simulink model "XY_2mm_accelcontrol"  (R2023a)
settings: Solver=ode1  StartTime=0.0  StopTime=inf  FixedStep=0.001  RelTol=1e-3  EnableMultiTasking=on
PostLoadFcn:
  | , if any(exist('dsrtsu_mdlpostloadfcn', 'file') ~= 0), dsrtsu_mdlpostloadfcn('Execute', bdroot); end,
InitFcn:
  | , if any(exist('rtifpga_mdlclblib', 'file') ~= 0), rtifpga_mdlclblib('Init', bdroot); end,
  | [b,a] = butter(6,0.6)
  | N_coils = 6
  | % Load mean voltage needed for stationary levitation at "center" for the ML model's given dataset
  | load("D:\Maglev_Project\00_WORKSTATION\MATLAB Training\alldata.mat","Vmean_raw")
  | tic
model workspace (MAT data in the model file):
  Iters = 5
  N_coils = 6
  fatness_default = 1
  running = 0
  z0_default = 0.080001
undefined symbols (not defined in the file or in its folder): a, b, DiscIntNeverNeededParam, Vmean_raw
libraries: neural x15, simulink x8, commfilt2 x7, dspstat3 x4, rti2004lib x3, rtilibm x1
(part 2 of 3)

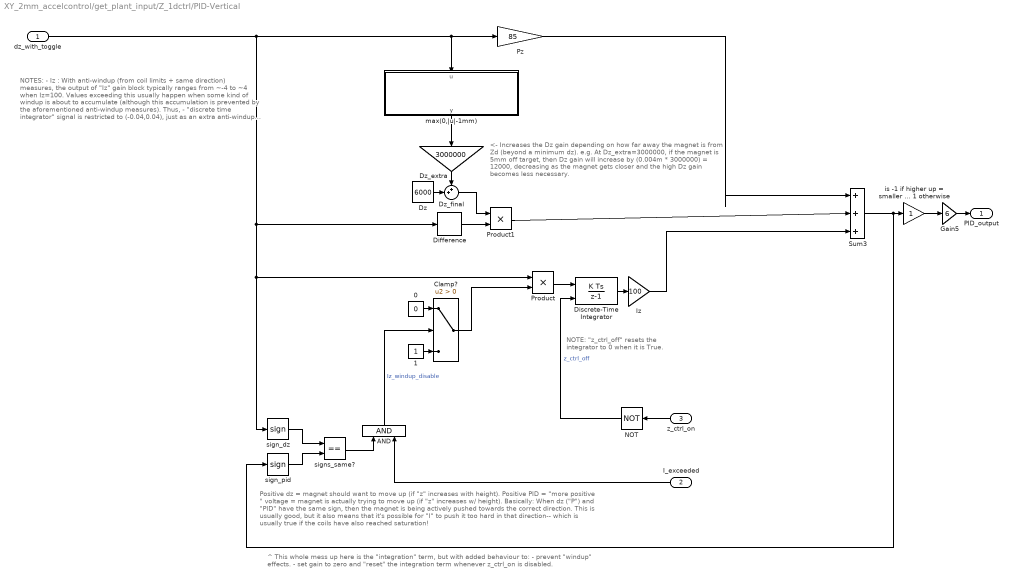
== system XY_2mm_accelcontrol/get_plant_input/Z_1dctrl/PID-Vertical ==
  note: <- Increases the Dz gain depending on how far away the magnet is from Zd (beyond a minimum dz).
      | e.g. At Dz_extra=3000000, if the magnet is 5mm off target, then Dz gain will increase by (0.004m * 3000000) = 12000, decreasing as the magnet gets closer and the high Dz gain becomes less necessary.
  note: NOTE: "z_ctrl_off" resets the integrator to 0 when it is True.
  note: NOTES:
      | - Iz : With anti-windup (from coil limits + same direction) measures, the output of "Iz" gain block typically ranges from ~-4 to ~4 when Iz=100. Values exceeding this usually happen when some kind of windup is about to accumulate (although this accumulation is prevented by the aforementioned anti-windup measures).
      | Thus,
      | - "discrete time integrator" signal is restricted to (-0.04,0.04), just as an extra anti-windup measure.
      | - Also, the integral resets while z-control is disabled.
  note: ^ This whole mess up here is the "integration" term, but with added behaviour to:
      | - prevent "windup" effects.
      | - set gain to zero and "reset" the integration term whenever z_ctrl_on is disabled.
  note: Positive dz = magnet should want to move up (if "z" increases with height).
      | Positive PID = "more positive " voltage = magnet is actually trying to move up (if "z" increases w/ height).
      |
      | Basically: When dz ("P") and "PID" have the same sign, then the magnet is being actively pushed towards the correct direction. This is usually good, but it also means that it's possible for "I" to push it too hard in that direction-- which is usually true if the coils have also reached saturation!
  dz_with_toggle : Inport
  I_exceeded : Inport  Port=2
  z_ctrl_on : Inport  Port=3
  0 : Constant  Value=0
  1 : Constant
  AND : Logic  AllPortsSameDT=off  OutDataTypeStr=boolean
  Clamp? : Switch  Criteria=u2 > Threshold  SaturateOnIntegerOverflow=off  InputSameDT=off
  Difference : simulink/Discrete/Difference  ICPrevInput=0.0  OutMin=[]  OutMax=[]  OutDataType=fixdt(1, 16)  OutScaling=2^-10  DoSatur=off
  Discrete-Time Integrator : DiscreteIntegrator  ExternalReset=sampled level  SampleTime=-1  LimitOutput=on  UpperSaturationLimit=0.04  LowerSaturationLimit=-0.04  ICPrevOutput=DiscIntNeverNeededParam  ICPrevScaledInput=DiscIntNeverNeededParam
  Dz : Constant  Value=6000
  Dz_extra : Gain  Gain=3000000
  Dz_final : Sum  Inputs=++|
  Gain5 : Gain  Gain=6
  Iz : Gain  Gain=100
  NOT : Logic  Operator=NOT  AllPortsSameDT=off  OutDataTypeStr=boolean
  Product : Product
  Product1 : Product
  Pz : Gain  Gain=85
  Sum3 : Sum  Inputs=|+++
  "is -1 if higher up = smaller z, 1 otherwise" : Gain
  max(0,|u|-1mm) : MATLAB Function  TreatAsAtomicUnit=on
  sign_dz : Signum
  sign_pid : Signum
  signs_same? : RelationalOperator  Operator===  OutDataTypeStr=boolean  RndMeth=Simplest  InputSameDT=off
  PID_output : Outport
  wires:
  Pz/1 -> Sum3/1
  Difference/1 -> Product1/2
  Product1/1 -> Sum3/2
  Sum3/1 -> sign_pid/1, "is -1 if higher up = smaller z, 1 otherwise"/1
  "is -1 if higher up = smaller z, 1 otherwise"/1 -> Gain5/1
  Gain5/1 -> PID_output/1
  0/1 -> Clamp?/1
  Discrete-Time Integrator/1 -> Iz/1
  Clamp?/1 -> Product/2
  Product/1 -> Discrete-Time Integrator/1
  1/1 -> Clamp?/3
  sign_dz/1 -> signs_same?/1
  sign_pid/1 -> signs_same?/2
  signs_same?/1 -> AND/1
  I_exceeded/1 -> AND/2
  AND/1 -> Clamp?/2  "Iz_windup_disable"
  z_ctrl_on/1 -> NOT/1
  NOT/1 -> Discrete-Time Integrator/2  "z_ctrl_off"
  Iz/1 -> Sum3/3
  dz_with_toggle/1 -> Difference/1, sign_dz/1, Product/1, max(0,|u|-1mm)/1(u), Pz/1
  Dz/1 -> Dz_final/2
  max(0,|u|-1mm)/1(y) -> Dz_extra/1
  Dz_extra/1 -> Dz_final/1
  Dz_final/1 -> Product1/1

== system XY_2mm_accelcontrol/get_plant_input/acceleration_to_I_ratio/Actually apply voltages ==
  note: Behaviour summary:
      | (HOLD, START):
      | 	(ON, ON)	- Voltage ratio is updated, but then stays constant
      | 	(ON, OFF)	- Voltage ratio cannot change
      |
      | 	(OFF, ON)	- Voltage ratio is continually updated to maintain input acceleration
      | 	(OFF, OFF)	- Voltage ratio cannot change
  note: User inputs:
      | “Hold ratio”
      | ON: Voltage ratio is held, so magnet will (ideally) accelerate as specified VERY BRIEFLY before settling at a Bmax point
      | OFF: Voltage ratio is dynamically adjusted to maintain the input acceleration (i.e. magnet will speed up endlessly)
      |
      | "Start acceleration" (HOLD)
      | ON: Voltage ratio is allowed to change while pressed
      | OFF: Voltage ratio is NOT allowed to change
  Voltages : Inport
  Hold ratio : Constant
  Start Acceleration : Constant  Value=0
  allow_voltage_update : Subsystem
  voltages_updated : Subsystem  TreatAsAtomicUnit=on
  Out1 : Outport
  wires:
  voltages_updated/1(voltages_updated) -> Out1/1
  Hold ratio/1 -> allow_voltage_update/1(Hold)
  Voltages/1 -> voltages_updated/1(voltages)
  Start Acceleration/1 -> allow_voltage_update/2(Start)
  allow_voltage_update/1(allow_voltage_update) -> voltages_updated/Enable

== system XY_2mm_accelcontrol/get_plant_input/acceleration_to_I_ratio/Make ratios add up to 1 ==
  note: Modified coil ratio distribution is ""normalized"" (NOT vector normalization) such that its sum equals 1.
  Voltages : Inport
  Divide : Product  Inputs=*/
  Sum of Elements : Sum  Inputs=+
  Voltage_ratio : Outport
  wires:
  Voltages/1 -> Sum of Elements/1, Divide/1
  Sum of Elements/1 -> Divide/2
  Divide/1 -> Voltage_ratio/1

== system XY_2mm_accelcontrol/get_plant_input/acceleration_to_I_ratio/Voltages from ML ==
  note: Current ML model (" DEFAULT_goodunits_filtervolts_TEMP ") inputs XY position (in mm) and a desired XY acceleration (in mm/s/s), and outputs final input voltages (i.e. voltages fed into amplifier) in V.
  xy_acc_mmss : Inport
  xy_mm : Inport  Port=2
  Function Fitting Neural Network : Subsystem
      mask help: Function Fitting Neural Network
      mask Display: e = 0.06;c1 = [120 150 230]/255;c2 = ([120 150 230]+0)/383;c3 = ([120 150 230]+128)/383;patch([0 1 1 0],[0 0 1 1],c1);patch([0 1 1 1-e 1-e 0+e],[0 0 1 1-e 0+e 0+e],c2);patch([0 0 1 1-e 0+e 0+e],[0 1 1 1-e 1-e 0+e],c3);plot([0 1 1 0 0],[0 0 1 1 0]);fprintf('NNET');port_label('input',1,' Input');port_label('output',1,'Output ');
  Mux : Mux  Inputs=2
  Sum : Sum  Inputs=|++
  Vmean : Constant  Value=Vmean_raw
  Voltages : Outport
  wires:
  xy_acc_mmss/1 -> Mux/2
  Vmean/1 -> Sum/2
  Function Fitting Neural Network/1(Output) -> Sum/1
  Sum/1 -> Voltages/1
  xy_mm/1 -> Mux/1
  Mux/1 -> Function Fitting Neural Network/1(Input)

== system XY_2mm_accelcontrol/get_plant_input/choose_Z_d_temp/istrue_for_X_time ==
  note: When is nonzero or true , the integrator accumulates by 1 per cycle. The counter stops and resets to 0 whenever input==0. Once the integrator crosses a certain threshold , the subsystem outputs 1 (0 otherwise). (In other words, it's just a timer for how long " logical(input) == 1 " has been maintained.)
      |
      | Basically, this subsystem outputs 1 if the input signal has been nonzero for X amount of time. Otherwise, it outputs 0.
  input : Inport
  Data Type Conversion : DataTypeConversion  OutDataTypeStr=boolean  SaturateOnIntegerOverflow=off  RndMeth=Floor
  Discrete-Time Accumulator (ms) : DiscreteIntegrator  IntegratorMethod=Accumulation: Forward Euler  ExternalReset=sampled level  SampleTime=-1  OutDataTypeStr=double  ICPrevOutput=DiscIntNeverNeededParam  ICPrevScaledInput=DiscIntNeverNeededParam
  GreaterThan : RelationalOperator  Operator=>  OutDataTypeStr=boolean  RndMeth=Simplest  InputSameDT=off
  NOT : Logic  Operator=NOT  AllPortsSameDT=off  OutDataTypeStr=boolean
  threshold_ms : Constant  Value=500
  input_held : Outport
  wires:
  input/1 -> Data Type Conversion/1
  Discrete-Time Accumulator (ms)/1 -> GreaterThan/1
  threshold_ms/1 -> GreaterThan/2
  NOT/1 -> Discrete-Time Accumulator (ms)/2
  GreaterThan/1 -> input_held/1
  Data Type Conversion/1 -> NOT/1, Discrete-Time Accumulator (ms)/1

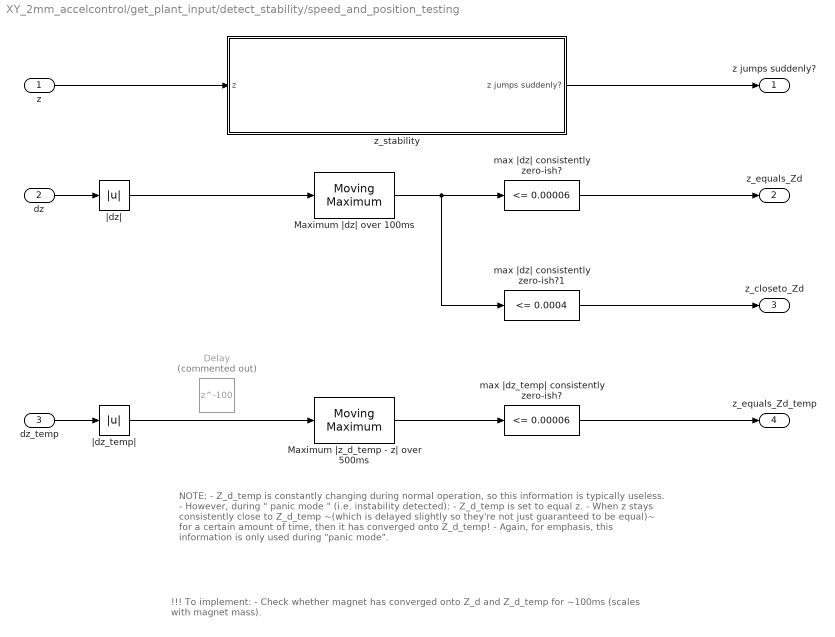
== system XY_2mm_accelcontrol/get_plant_input/detect_stability/speed_and_position_testing ==
  note: !!! To implement:
      | - Check whether magnet has converged onto Z_d and Z_d_temp for ~100ms (scales with magnet mass).
  note: NOTE:
      | - Z_d_temp is constantly changing during normal operation, so this information is typically useless.
      | - However, during " panic mode " (i.e. instability detected):
      | - Z_d_temp is set to equal z.
      | - When z stays consistently close to Z_d_temp ~(which is delayed slightly so they're not just
      | guaranteed to be equal)~ for a certain amount of time, then it has converged onto Z_d_temp!
      | - Again, for emphasis, this information is only used during "panic mode".
  z : Inport
  dz : Inport  Port=2
  dz_temp : Inport  Port=3
  Delay : Delay  Commented=on  DelayLength=100
  Maximum |dz| over 100ms : dspstat3/Moving Maximum  SpecifyWindowLength=on  WindowLength=100  SimulateUsing=Code generation
  Maximum |z_d_temp - z| over 500ms : dspstat3/Moving Maximum  SpecifyWindowLength=on  WindowLength=500  SimulateUsing=Code generation
  max |dz_temp| consistently zero-ish? : simulink/Logic and Bit Operations/Compare To Constant  relop=<=  const=0.00006  OutDataTypeStr=boolean
  max |dz| consistently zero-ish? : simulink/Logic and Bit Operations/Compare To Constant  relop=<=  const=0.00006  OutDataTypeStr=boolean
  max |dz| consistently zero-ish?1 : simulink/Logic and Bit Operations/Compare To Constant  relop=<=  const=0.0004  OutDataTypeStr=boolean
  z_stability : Subsystem
  |dz_temp| : Abs  SaturateOnIntegerOverflow=off
  |dz| : Abs  SaturateOnIntegerOverflow=off
  z jumps suddenly? : Outport
  z_equals_Zd : Outport  Port=2
  z_closeto_Zd : Outport  Port=3
  z_equals_Zd_temp : Outport  Port=4
  wires:
  |dz|/1 -> Maximum |dz| over 100ms/1
  max |dz| consistently zero-ish?/1 -> z_equals_Zd/1
  dz/1 -> |dz|/1
  Maximum |z_d_temp - z| over 500ms/1 -> max |dz_temp| consistently zero-ish?/1
  max |dz_temp| consistently zero-ish?/1 -> z_equals_Zd_temp/1
  dz_temp/1 -> |dz_temp|/1
  |dz_temp|/1 -> Maximum |z_d_temp - z| over 500ms/1
  z/1 -> z_stability/1(z)
  max |dz| consistently zero-ish?1/1 -> z_closeto_Zd/1
  Maximum |dz| over 100ms/1 -> max |dz| consistently zero-ish?1/1, max |dz| consistently zero-ish?/1
  z_stability/1(z jumps suddenly?) -> z jumps suddenly?/1

== system XY_2mm_accelcontrol/plant/Position Determination1/10ms mean x ==
  note: NOTE: Sensor readings fluctuate over a peak-to-peak amplitude of about 4.5e-5 m, over a period of almost exactly 10ms.
      |
      | 08/14/23: See how it improves if I only consider the mean signal over 10ms!
  In1 : Inport
  ave signal : Product  Inputs=*/
  integration window (samples) : Constant  Value=10
  sum of signal over short time : commfilt2/Windowed Integrator  integperiod=10  InputProcessing=Columns as channels (frame based)  roundingMode=Floor  overflowMode=off  coeffDataTypeStr=Inherit: Same word length as input  coeffMin=[]  coeffMax=[]  coeffLastDataTypeStr=Inherit: Same word length as input  accumDataTypeStr=Inherit: Same as product output  accumLastDataTypeStr=Inherit: Same as product output  outputDataTypeStr=Inherit: Same as accumulator  outputMin=[]  outputMax=[]  outputLastDataTypeStr=Inherit: Same as accumulator
  X(m) : Outport
  wires:
  sum of signal over short time/1 -> ave signal/1
  In1/1 -> sum of signal over short time/1
  integration window (samples)/1 -> ave signal/2
  ave signal/1 -> X(m)/1

== system XY_2mm_accelcontrol/plant/Position Determination1/10ms mean y ==
  note: NOTE: Sensor readings fluctuate over a peak-to-peak amplitude of about 4.5e-5 m, over a period of almost exactly 10ms.
      |
      | 08/14/23: See how it improves if I only consider the mean signal over 10ms!
  In1 : Inport
  ave signal : Product  Inputs=*/
  integration window (samples) : Constant  Value=10
  sum of signal over short time : commfilt2/Windowed Integrator  integperiod=10  InputProcessing=Columns as channels (frame based)  roundingMode=Floor  overflowMode=off  coeffDataTypeStr=Inherit: Same word length as input  coeffMin=[]  coeffMax=[]  coeffLastDataTypeStr=Inherit: Same word length as input  accumDataTypeStr=Inherit: Same as product output  accumLastDataTypeStr=Inherit: Same as product output  outputDataTypeStr=Inherit: Same as accumulator  outputMin=[]  outputMax=[]  outputLastDataTypeStr=Inherit: Same as accumulator
  Y(m) : Outport
  wires:
  sum of signal over short time/1 -> ave signal/1
  In1/1 -> sum of signal over short time/1
  integration window (samples)/1 -> ave signal/2
  ave signal/1 -> Y(m)/1

== system XY_2mm_accelcontrol/plant/Position Determination1/10ms mean z ==
  note: NOTE: Sensor readings fluctuate over a peak-to-peak amplitude of about 4.5e-5 m, over a period of almost exactly 10ms.
      |
      | 08/14/23: See how it improves if I only consider the mean signal over 10ms!
  In1 : Inport
  ave signal : Product  Inputs=*/
  integration window (samples) : Constant  Value=10
  sum of signal over short time : commfilt2/Windowed Integrator  integperiod=10  InputProcessing=Columns as channels (frame based)  roundingMode=Floor  overflowMode=off  coeffDataTypeStr=Inherit: Same word length as input  coeffMin=[]  coeffMax=[]  coeffLastDataTypeStr=Inherit: Same word length as input  accumDataTypeStr=Inherit: Same as product output  accumLastDataTypeStr=Inherit: Same as product output  outputDataTypeStr=Inherit: Same as accumulator  outputMin=[]  outputMax=[]  outputLastDataTypeStr=Inherit: Same as accumulator
  Z(m) : Outport
  wires:
  sum of signal over short time/1 -> ave signal/1
  In1/1 -> sum of signal over short time/1
  integration window (samples)/1 -> ave signal/2
  ave signal/1 -> Z(m)/1

== system XY_2mm_accelcontrol/plant/Position Determination1/XY position Calculation ==
  note: !!MODIFIED!!
      | Before: "X_p, Y_p = Head2_read, Head3_read - radius_m".
      | After: "Head2_p, Head3_p = Head2_read, Head3_read + radius_m".
  note: Laser sensors output a voltage in [-10,10]V, proportional to the detected object's position-- which ranges from 0mm (up, given by 10V) to 40mm (down, given by -10V). Size of the object is not taken into account.
  Head II (Voltage) : Inport
  Head III (Voltage) : Inport  Port=2
  diameter_m : Inport  Port=3
  Gain : Gain  Gain=1/2
  Gain2 : Gain  Gain=2/1000
  Gain4 : Gain  Gain=2/1000
  Mux : Mux  Inputs=2
  Sum : Sum  Inputs=|++
  Sum1 : Sum  Inputs=++|
  X_m : Fcn  Expr=(u(1)+u(2))*sin(pi/4)
  Y_m : Fcn  Expr=(u(1)-u(2))*sin(pi/4)
  X_Position(m) : Outport
  Y_Position(m) : Outport  Port=2
  wires:
  Head III (Voltage)/1 -> Gain4/1
  Y_m/1 -> Y_Position(m)/1
  X_m/1 -> X_Position(m)/1
  Head II (Voltage)/1 -> Gain2/1
  Mux/1 -> Y_m/1, X_m/1
  Sum1/1 -> Mux/2  "Head3_p"
  Gain4/1 -> Sum1/2
  Sum/1 -> Mux/1  "Head2_p"
  Gain/1 -> Sum1/1, Sum/2  "radius_m"
  Gain2/1 -> Sum/1
  diameter_m/1 -> Gain/1

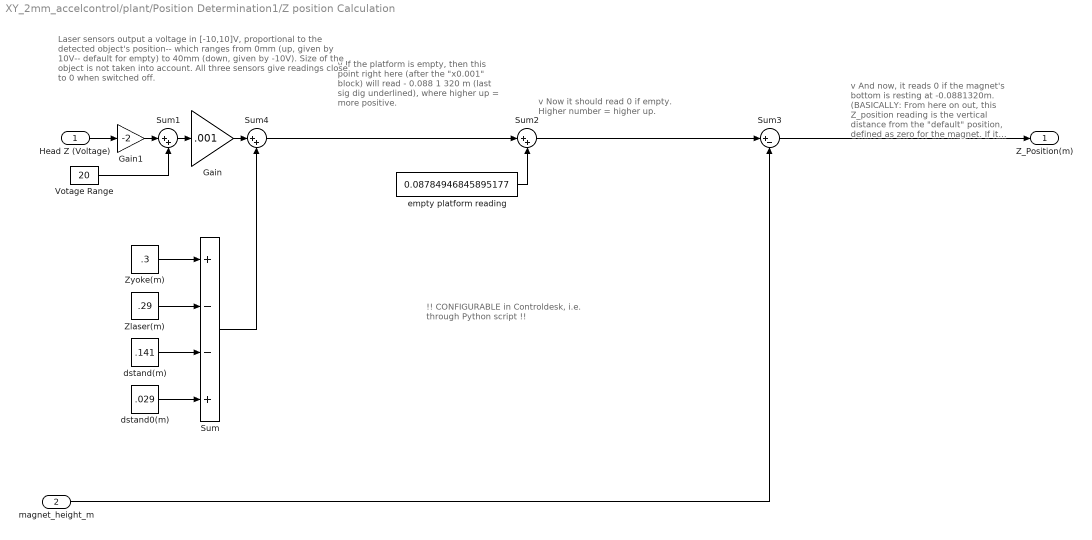
== system XY_2mm_accelcontrol/plant/Position Determination1/Z position Calculation ==
  note: v If the platform is empty, then this point right here (after the "x0.001" block) will read - 0.088 1 320 m (last sig dig underlined), where higher up = more positive.
  note: Laser sensors output a voltage in [-10,10]V, proportional to the detected object's position-- which ranges from 0mm (up, given by 10V-- default for empty) to 40mm (down, given by -10V). Size of the object is not taken into account.
      | All three sensors give readings close to 0 when switched off.
  note: v Now it should read 0 if empty.
      | Higher number = higher up.
  note: v And now, it reads 0 if the magnet's bottom is resting at -0.0881320m.
      |
      | (BASICALLY: From here on out, this Z_position reading is the vertical distance from the "default" position, defined as zero for the magnet. If it reads something significantly different from 0, then double check the magnet height.)
  note: !! CONFIGURABLE in Controldesk, i.e. through Python script !!
  Head Z (Voltage) : Inport
  magnet_height_m : Inport  Port=2
  Gain : Gain  Gain=.001
  Gain1 : Gain  Gain=-2
  Sum : Sum  Inputs=+--+
  Sum1 : Sum  Inputs=|++
  Sum2 : Sum  Inputs=|++
  Sum3 : Sum  Inputs=|+-
  Sum4 : Sum  Inputs=|++
  Votage Range : Constant  Value=20
  Zlaser(m) : Constant  Value=.29
  Zyoke(m) : Constant  Value=.3
  dstand(m) : Constant  Value=.141
  dstand0(m) : Constant  Value=.029
  empty platform reading : Constant  Value=0.08784946845895177
  Z_Position(m) : Outport
  wires:
  Sum2/1 -> Sum3/1
  Head Z (Voltage)/1 -> Gain1/1
  Sum/1 -> Sum4/2
  Sum1/1 -> Gain/1
  Votage Range/1 -> Sum1/2
  Gain1/1 -> Sum1/1
  Zlaser(m)/1 -> Sum/2
  Zyoke(m)/1 -> Sum/1
  dstand(m)/1 -> Sum/3
  dstand0(m)/1 -> Sum/4
  magnet_height_m/1 -> Sum3/2
  Sum4/1 -> Sum2/1
  Gain/1 -> Sum4/1
  empty platform reading/1 -> Sum2/2
  Sum3/1 -> Z_Position(m)/1

== system XY_2mm_accelcontrol/RTI Data/RTI Data Store/RTI Data Store/RTI Data Store ==
  RTI Data Store : Subsystem  mask(RTI_DATA_STORE){}
      mask help:
      | RTI Data Store Block. This block is used by RTI to store internal model dependent data. Deleting this block will result in data loss.
      |
      | NEVER DELETE, COPY, OR MODIFY THIS BLOCK!
      mask Help:
      | RTI Data Store Block. This block is used by RTI to store internal model dependent data. Deleting this block will result in data loss.
      | 
      | NEVER DELETE, COPY, OR MODIFY THIS BLOCK!
      mask Display: text(0.5, 0.5, ' ', 'HorizontalAlignment', 'center');

== system XY_2mm_accelcontrol/get_plant_input/acceleration_to_I_ratio/Actually apply voltages/allow_voltage_update ==
  Hold : Inport
  Start : Inport  Port=2
  AND : Logic  AllPortsSameDT=off  OutDataTypeStr=boolean
  NOT : Logic  Operator=NOT  IconShape=distinctive  AllPortsSameDT=off  OutDataTypeStr=boolean
  OR : Logic  Operator=OR  AllPortsSameDT=off  OutDataTypeStr=boolean
  was Start just enabled : Subsystem
  allow_voltage_update : Outport
  wires:
  Start/1 -> was Start just enabled/1(Start), AND/2
  Hold/1 -> NOT/1
  AND/1 -> allow_voltage_update/1
  was Start just enabled/1(just_activated) -> OR/2
  OR/1 -> AND/1
  NOT/1 -> OR/1

== system XY_2mm_accelcontrol/get_plant_input/acceleration_to_I_ratio/Actually apply voltages/voltages_updated ==
  voltages : Inport
  Enable : EnablePort
  voltages_updated : Outport
  wires:
  voltages/1 -> voltages_updated/1

== system XY_2mm_accelcontrol/get_plant_input/acceleration_to_I_ratio/Voltages from ML/Function Fitting Neural Network ==
  Input : Inport  PortDimensions=4
      mask Display: e = 0.06;c1 = [120 230 180]/255;c2 = ([120 230 180]+0)/(256+128);c3 = ([120 230 180]+128)/(256+128);patch([0 1 1 0],[0 0 1 1],c1);patch([0 1 1 1-e 1-e 0+e],[0 0 1 1-e 0+e 0+e],c2);patch([0 0 1 1-e 0+e 0+e],[0 1 1 1-e 1-e 0+e],c3);plot([0 1 1 0 0],[0 0 1 1 0]);
  Layer 1 : Subsystem
      mask Display: e = 0.06;c1 = [120 150 230]/255;c2 = ([120 150 230]+0)/383;c3 = ([120 150 230]+128)/383;patch([0 1 1 0],[0 0 1 1],c1);patch([0 1 1 1-e 1-e 0+e],[0 0 1 1-e 0+e 0+e],c2);patch([0 0 1 1-e 0+e 0+e],[0 1 1 1-e 1-e 0+e],c3);plot([0 1 1 0 0],[0 0 1 1 0]);
  Layer 2 : Subsystem
      mask Display: e = 0.06;c1 = [120 150 230]/255;c2 = ([120 150 230]+0)/383;c3 = ([120 150 230]+128)/383;patch([0 1 1 0],[0 0 1 1],c1);patch([0 1 1 1-e 1-e 0+e],[0 0 1 1-e 0+e 0+e],c2);patch([0 0 1 1-e 0+e 0+e],[0 1 1 1-e 1-e 0+e],c3);plot([0 1 1 0 0],[0 0 1 1 0]);
  Process Input 1 : Subsystem
      mask Display: e = 0.06;c1 = [120 150 230]/255;c2 = ([120 150 230]+0)/383;c3 = ([120 150 230]+128)/383;patch([0 1 1 0],[0 0 1 1],c1);patch([0 1 1 1-e 1-e 0+e],[0 0 1 1-e 0+e 0+e],c2);patch([0 0 1 1-e 0+e 0+e],[0 1 1 1-e 1-e 0+e],c3);plot([0 1 1 0 0],[0 0 1 1 0]);
  Process Output 1 : Subsystem
      mask Display: e = 0.06;c1 = [120 150 230]/255;c2 = ([120 150 230]+0)/383;c3 = ([120 150 230]+128)/383;patch([0 1 1 0],[0 0 1 1],c1);patch([0 1 1 1-e 1-e 0+e],[0 0 1 1-e 0+e 0+e],c2);patch([0 0 1 1-e 0+e 0+e],[0 1 1 1-e 1-e 0+e],c3);plot([0 1 1 0 0],[0 0 1 1 0]);
  Output : Outport  InitialOutput=[0;0;0;0;0;0]
      mask Display: e = 0.06;c1 = [120 230 180]/255;c2 = ([120 230 180]+0)/(256+128);c3 = ([120 230 180]+128)/(256+128);patch([0 1 1 0],[0 0 1 1],c1);patch([0 1 1 1-e 1-e 0+e],[0 0 1 1-e 0+e 0+e],c2);patch([0 0 1 1-e 0+e 0+e],[0 1 1 1-e 1-e 0+e],c3);plot([0 1 1 0 0],[0 0 1 1 0]);
  wires:
  Input/1 -> Process Input 1/1(x)
  Process Output 1/1(y) -> Output/1
  Process Input 1/1(p) -> Layer 1/1("p{1}")
  Layer 1/1("a{1}") -> [feedback1]
  [feedback1] -> Layer 2/1("a{1} ")
  Layer 2/1("a{2}") -> Process Output 1/1(a)

== system XY_2mm_accelcontrol/get_plant_input/detect_stability/speed_and_position_testing/z_stability ==
  note: NOTE:
      | When Zd changes, the speed peaks spike up from ~5e-7m/s to around ~2e-5 m/s.
      |
      | When the magnet struggles to converge, the speed peaks spike up to ~1e-5 or more.
      |
      | Thus: 0.5e-5 m/s seems to be a good line beyond which speed peaks indicate either intentional vertical movement OR struggle/failure to converge onto Zd. When this occurs will be tracked using a moving maximum over some short timeframe (~100ms?).
      |
      | ** The above is WITH "z" being the 10ms average of the raw signal. Changing this may require recalibration of this speed threshold. **
  z : Inport
  Abs : Abs  Commented=on  SaturateOnIntegerOverflow=off
  Highest z in past 25ms : dspstat3/Moving Maximum  Commented=on  SpecifyWindowLength=on  WindowLength=25  SimulateUsing=Code generation
  Lowest z in past 25ms : dspstat3/Moving Minimum  Commented=on  SpecifyWindowLength=on  WindowLength=25  SimulateUsing=Code generation
  Sum : Sum  Commented=on  Inputs=|+-|
  ave z : Product  Inputs=*/
  average |z - z_prev|/dt (m/ms) too high? : simulink/Logic and Bit Operations/Compare To Constant  relop=>=  const=0.5e-5  OutDataTypeStr=boolean
  integration window (samples)2 : Constant  Value=10
  sum of z over 10ms1 : commfilt2/Windowed Integrator  integperiod=10  InputProcessing=Columns as channels (frame based)  roundingMode=Floor  overflowMode=off  coeffDataTypeStr=Inherit: Same word length as input  coeffMin=[]  coeffMax=[]  coeffLastDataTypeStr=Inherit: Same word length as input  accumDataTypeStr=Inherit: Same as product output  accumLastDataTypeStr=Inherit: Same as product output  outputDataTypeStr=Inherit: Same as accumulator  outputMin=[]  outputMax=[]  outputLastDataTypeStr=Inherit: Same as accumulator
  z - z_previous : simulink/Discrete/Difference  ICPrevInput=0.0  OutMin=[]  OutMax=[]  OutDataType=fixdt(1, 16)  OutScaling=2^-10  DoSatur=off
  z jumps by more than 0.15mm in 25ms? : simulink/Logic and Bit Operations/Compare To Constant  Commented=on  relop=>=  const=0.00015  OutDataTypeStr=boolean
  |z - z_previous| : Abs  SaturateOnIntegerOverflow=off
  z jumps suddenly? : Outport
  wires:
  Abs/1 -> z jumps by more than 0.15mm in 25ms?/1
  z/1 -> sum of z over 10ms1/1
  Highest z in past 25ms/1 -> Sum/2
  Sum/1 -> Abs/1
  Lowest z in past 25ms/1 -> Sum/1
  z jumps by more than 0.15mm in 25ms?/1 -> ?
  integration window (samples)2/1 -> ave z/2
  sum of z over 10ms1/1 -> ave z/1
  z - z_previous/1 -> |z - z_previous|/1
  ave z/1 -> z - z_previous/1
  |z - z_previous|/1 -> average |z - z_prev|/dt (m/ms) too high?/1
  average |z - z_prev|/dt (m/ms) too high?/1 -> z jumps suddenly?/1

== system XY_2mm_accelcontrol/RTI Data/RTI Data Store/RTI Data Store/RTI Data Store/RTI Data Store ==

== system XY_2mm_accelcontrol/get_plant_input/acceleration_to_I_ratio/Actually apply voltages/allow_voltage_update/was Start just enabled ==
  Start : Inport
  Delay One Step : Delay  DelayLength=1
  Greaterthan : RelationalOperator  Operator=>  OutDataTypeStr=boolean  RndMeth=Simplest  InputSameDT=off
  just_activated : Outport
  wires:
  Start/1 -> Greaterthan/1, Delay One Step/1
  Delay One Step/1 -> Greaterthan/2
  Greaterthan/1 -> just_activated/1

== system XY_2mm_accelcontrol/get_plant_input/acceleration_to_I_ratio/Voltages from ML/Function Fitting Neural Network/Layer 1 ==
  "p{1}" : Inport  PortDimensions=4
      mask Display: e = 0.06;c1 = [120 230 180]/255;c2 = ([120 230 180]+0)/(256+128);c3 = ([120 230 180]+128)/(256+128);patch([0 1 1 0],[0 0 1 1],c1);patch([0 1 1 1-e 1-e 0+e],[0 0 1 1-e 0+e 0+e],c2);patch([0 0 1 1-e 0+e 0+e],[0 1 1 1-e 1-e 0+e],c3);plot([0 1 1 0 0],[0 0 1 1 0]);
  Delays 1 : Subsystem
      mask Display: e = 0.06;c1 = [120 150 230]/255;c2 = ([120 150 230]+0)/383;c3 = ([120 150 230]+128)/383;patch([0 1 1 0],[0 0 1 1],c1);patch([0 1 1 1-e 1-e 0+e],[0 0 1 1-e 0+e 0+e],c2);patch([0 0 1 1-e 0+e 0+e],[0 1 1 1-e 1-e 0+e],c3);plot([0 1 1 0 0],[0 0 1 1 0]);disp('0');
  "IW{1,1}" : Subsystem
      mask Display: e = 0.06;c1 = [120 150 230]/255;c2 = ([120 150 230]+0)/383;c3 = ([120 150 230]+128)/383;patch([0 1 1 0],[0 0 1 1],c1);patch([0 1 1 1-e 1-e 0+e],[0 0 1 1-e 0+e 0+e],c2);patch([0 0 1 1-e 0+e 0+e],[0 1 1 1-e 1-e 0+e],c3);plot([0 1 1 0 0],[0 0 1 1 0]);disp('W');
  "b{1}" : Constant  Value=[0.2425447899040890920030477673208224587142467498779296875;0.99314547038972278425461581718991510570049285888671875;-0.328895397762378915995640227265539579093456268310546875;-1.38849780916554177423449800699017941951751708984375;-0.26530583823266418175279568458790890872478485107421875]
      mask Display: e = 0.06;c1 = [120 150 230]/255;c2 = ([120 150 230]+0)/383;c3 = ([120 150 230]+128)/383;patch([0 1 1 0],[0 0 1 1],c1);patch([0 1 1 1-e 1-e 0+e],[0 0 1 1-e 0+e 0+e],c2);patch([0 0 1 1-e 0+e 0+e],[0 1 1 1-e 1-e 0+e],c3);plot([0 1 1 0 0],[0 0 1 1 0]);disp('b');
  netsum : Sum  Inputs=2  InputSameDT=on  SaturateOnIntegerOverflow=on  OutDataTypeStr=Inherit: Same as first input
      mask Display: e = 0.06;c1 = [120 150 230]/255;c2 = ([120 150 230]+0)/383;c3 = ([120 150 230]+128)/383;patch([0 1 1 0],[0 0 1 1],c1);patch([0 1 1 1-e 1-e 0+e],[0 0 1 1-e 0+e 0+e],c2);patch([0 0 1 1-e 0+e 0+e],[0 1 1 1-e 1-e 0+e],c3);plot([0 1 1 0 0],[0 0 1 1 0]);disp('+');
  tansig : neural/Transfer Functions/tansig
  "a{1}" : Outport  InitialOutput=[0;0;0;0;0]
      mask Display: e = 0.06;c1 = [120 230 180]/255;c2 = ([120 230 180]+0)/(256+128);c3 = ([120 230 180]+128)/(256+128);patch([0 1 1 0],[0 0 1 1],c1);patch([0 1 1 1-e 1-e 0+e],[0 0 1 1-e 0+e 0+e],c2);patch([0 0 1 1-e 0+e 0+e],[0 1 1 1-e 1-e 0+e],c3);plot([0 1 1 0 0],[0 0 1 1 0]);
  wires:
  "p{1}"/1 -> Delays 1/1("p{1}")
  Delays 1/1("pd{1,1}") -> "IW{1,1}"/1("pd{1,1}")
  "IW{1,1}"/1("iz{1,1}") -> netsum/1
  "b{1}"/1 -> netsum/2
  netsum/1 -> tansig/1
  tansig/1 -> "a{1}"/1

== system XY_2mm_accelcontrol/get_plant_input/acceleration_to_I_ratio/Voltages from ML/Function Fitting Neural Network/Layer 2 ==
  "a{1} " : Inport  PortDimensions=5
      mask Display: e = 0.06;c1 = [120 230 180]/255;c2 = ([120 230 180]+0)/(256+128);c3 = ([120 230 180]+128)/(256+128);patch([0 1 1 0],[0 0 1 1],c1);patch([0 1 1 1-e 1-e 0+e],[0 0 1 1-e 0+e 0+e],c2);patch([0 0 1 1-e 0+e 0+e],[0 1 1 1-e 1-e 0+e],c3);plot([0 1 1 0 0],[0 0 1 1 0]);
  Delays 1 : Subsystem
      mask Display: e = 0.06;c1 = [120 150 230]/255;c2 = ([120 150 230]+0)/383;c3 = ([120 150 230]+128)/383;patch([0 1 1 0],[0 0 1 1],c1);patch([0 1 1 1-e 1-e 0+e],[0 0 1 1-e 0+e 0+e],c2);patch([0 0 1 1-e 0+e 0+e],[0 1 1 1-e 1-e 0+e],c3);plot([0 1 1 0 0],[0 0 1 1 0]);disp('0');
  "LW{2,1}" : Subsystem
      mask Display: e = 0.06;c1 = [120 150 230]/255;c2 = ([120 150 230]+0)/383;c3 = ([120 150 230]+128)/383;patch([0 1 1 0],[0 0 1 1],c1);patch([0 1 1 1-e 1-e 0+e],[0 0 1 1-e 0+e 0+e],c2);patch([0 0 1 1-e 0+e 0+e],[0 1 1 1-e 1-e 0+e],c3);plot([0 1 1 0 0],[0 0 1 1 0]);disp('W');
  "b{2}" : Constant  Value=[-1.3296693862343527126057551868143491446971893310546875;1.159994031312905793384970820625312626361846923828125;-0.97580089616446163969243343672133050858974456787109375;1.31789692191591267800276909838430583477020263671875;-1.1602838775240111868214398782583884894847869873046875;0.958380635005961156736020711832679808139801025390625]
      mask Display: e = 0.06;c1 = [120 150 230]/255;c2 = ([120 150 230]+0)/383;c3 = ([120 150 230]+128)/383;patch([0 1 1 0],[0 0 1 1],c1);patch([0 1 1 1-e 1-e 0+e],[0 0 1 1-e 0+e 0+e],c2);patch([0 0 1 1-e 0+e 0+e],[0 1 1 1-e 1-e 0+e],c3);plot([0 1 1 0 0],[0 0 1 1 0]);disp('b');
  netsum : Sum  Inputs=2  InputSameDT=on  SaturateOnIntegerOverflow=on  OutDataTypeStr=Inherit: Same as first input
      mask Display: e = 0.06;c1 = [120 150 230]/255;c2 = ([120 150 230]+0)/383;c3 = ([120 150 230]+128)/383;patch([0 1 1 0],[0 0 1 1],c1);patch([0 1 1 1-e 1-e 0+e],[0 0 1 1-e 0+e 0+e],c2);patch([0 0 1 1-e 0+e 0+e],[0 1 1 1-e 1-e 0+e],c3);plot([0 1 1 0 0],[0 0 1 1 0]);disp('+');
  purelin : neural/Transfer Functions/purelin
  "a{2}" : Outport  InitialOutput=[0;0;0;0;0;0]
      mask Display: e = 0.06;c1 = [120 230 180]/255;c2 = ([120 230 180]+0)/(256+128);c3 = ([120 230 180]+128)/(256+128);patch([0 1 1 0],[0 0 1 1],c1);patch([0 1 1 1-e 1-e 0+e],[0 0 1 1-e 0+e 0+e],c2);patch([0 0 1 1-e 0+e 0+e],[0 1 1 1-e 1-e 0+e],c3);plot([0 1 1 0 0],[0 0 1 1 0]);
  wires:
  "a{1} "/1 -> Delays 1/1("p{2}")
  Delays 1/1("pd{2,1}") -> "LW{2,1}"/1("ad{2,1}")
  "LW{2,1}"/1("lz{2,1}") -> netsum/1
  "b{2}"/1 -> netsum/2
  netsum/1 -> purelin/1
  purelin/1 -> "a{2}"/1

== system XY_2mm_accelcontrol/get_plant_input/acceleration_to_I_ratio/Voltages from ML/Function Fitting Neural Network/Process Input 1 ==
  x : Inport  PortDimensions=4
      mask Display: e = 0.06;c1 = [120 230 180]/255;c2 = ([120 230 180]+0)/(256+128);c3 = ([120 230 180]+128)/(256+128);patch([0 1 1 0],[0 0 1 1],c1);patch([0 1 1 1-e 1-e 0+e],[0 0 1 1-e 0+e 0+e],c2);patch([0 0 1 1-e 0+e 0+e],[0 1 1 1-e 1-e 0+e],c3);plot([0 1 1 0 0],[0 0 1 1 0]);
  mapminmax : neural/Processing Functions/mapminmax  xmin=[-2.57167105718465016650498000672;-2.87125469007469780180485940946;-2.90433201734715762398764127283;-2.05883064899576151418614244903]  xmax=[2.87985575989638808991344376409;2.86790458332340936209448045702;2.56774346823457033650583980489;1.64335200147816884452822705498]  ymin=-1  ymax=1
  p : Outport  PortDimensions=4
      mask Display: e = 0.06;c1 = [120 230 180]/255;c2 = ([120 230 180]+0)/(256+128);c3 = ([120 230 180]+128)/(256+128);patch([0 1 1 0],[0 0 1 1],c1);patch([0 1 1 1-e 1-e 0+e],[0 0 1 1-e 0+e 0+e],c2);patch([0 0 1 1-e 0+e 0+e],[0 1 1 1-e 1-e 0+e],c3);plot([0 1 1 0 0],[0 0 1 1 0]);
  wires:
  x/1 -> mapminmax/1
  mapminmax/1 -> p/1

== system XY_2mm_accelcontrol/get_plant_input/acceleration_to_I_ratio/Voltages from ML/Function Fitting Neural Network/Process Output 1 ==
  a : Inport  PortDimensions=6
      mask Display: e = 0.06;c1 = [120 230 180]/255;c2 = ([120 230 180]+0)/(256+128);c3 = ([120 230 180]+128)/(256+128);patch([0 1 1 0],[0 0 1 1],c1);patch([0 1 1 1-e 1-e 0+e],[0 0 1 1-e 0+e 0+e],c2);patch([0 0 1 1-e 0+e 0+e],[0 1 1 1-e 1-e 0+e],c3);plot([0 1 1 0 0],[0 0 1 1 0]);
  mapminmax_reverse : neural/Processing Functions/mapminmax_reverse  xmin=[-0.206749677587765523512075560575;-0.126838613782691428388815779726;-0.14642345900931330593408574714;-0.165157395081129698688471307833;-0.132595814081680613005786995018;-0.136116353697422670654404441848]  xmax=[0.0493857659930016790195139719799;0.0153151888660876811520950013801;0.0218207349655177018643570363565;0.0911455196341926787706455570515;0.0110405651020689943297981017167;0.0296361020287045640042578042994]  ymin=-1  ymax=1
  y : Outport  PortDimensions=6
      mask Display: e = 0.06;c1 = [120 230 180]/255;c2 = ([120 230 180]+0)/(256+128);c3 = ([120 230 180]+128)/(256+128);patch([0 1 1 0],[0 0 1 1],c1);patch([0 1 1 1-e 1-e 0+e],[0 0 1 1-e 0+e 0+e],c2);patch([0 0 1 1-e 0+e 0+e],[0 1 1 1-e 1-e 0+e],c3);plot([0 1 1 0 0],[0 0 1 1 0]);
  wires:
  a/1 -> mapminmax_reverse/1
  mapminmax_reverse/1 -> y/1

== system XY_2mm_accelcontrol/get_plant_input/acceleration_to_I_ratio/Voltages from ML/Function Fitting Neural Network/Layer 1/Delays 1 ==
  "p{1}" : Inport  PortDimensions=4
      mask Display: e = 0.06;c1 = [120 230 180]/255;c2 = ([120 230 180]+0)/(256+128);c3 = ([120 230 180]+128)/(256+128);patch([0 1 1 0],[0 0 1 1],c1);patch([0 1 1 1-e 1-e 0+e],[0 0 1 1-e 0+e 0+e],c2);patch([0 0 1 1-e 0+e 0+e],[0 1 1 1-e 1-e 0+e],c3);plot([0 1 1 0 0],[0 0 1 1 0]);
  mux : Mux  Inputs=1
      mask Display: e = 0.06;c1 = [120 150 230]/255;c2 = ([120 150 230]+0)/383;c3 = ([120 150 230]+128)/383;patch([0 1 1 0],[0 0 1 1],c1);patch([0 1 1 1-e 1-e 0+e],[0 0 1 1-e 0+e 0+e],c2);patch([0 0 1 1-e 0+e 0+e],[0 1 1 1-e 1-e 0+e],c3);plot([0 1 1 0 0],[0 0 1 1 0]);disp('Mux')
  "pd{1,1}" : Outport
      mask Display: e = 0.06;c1 = [120 230 180]/255;c2 = ([120 230 180]+0)/(256+128);c3 = ([120 230 180]+128)/(256+128);patch([0 1 1 0],[0 0 1 1],c1);patch([0 1 1 1-e 1-e 0+e],[0 0 1 1-e 0+e 0+e],c2);patch([0 0 1 1-e 0+e 0+e],[0 1 1 1-e 1-e 0+e],c3);plot([0 1 1 0 0],[0 0 1 1 0]);
  wires:
  "p{1}"/1 -> mux/1
  mux/1 -> "pd{1,1}"/1

== system XY_2mm_accelcontrol/get_plant_input/acceleration_to_I_ratio/Voltages from ML/Function Fitting Neural Network/Layer 1/IW{1,1} ==
  "pd{1,1}" : Inport  PortDimensions=4
      mask Display: e = 0.06;c1 = [120 230 180]/255;c2 = ([120 230 180]+0)/(256+128);c3 = ([120 230 180]+128)/(256+128);patch([0 1 1 0],[0 0 1 1],c1);patch([0 1 1 1-e 1-e 0+e],[0 0 1 1-e 0+e 0+e],c2);patch([0 0 1 1-e 0+e 0+e],[0 1 1 1-e 1-e 0+e],c3);plot([0 1 1 0 0],[0 0 1 1 0]);
  "IW{1,1}(1,:)'" : Constant  Value=[-0.186628540785822139014271670021116733551025390625;1.092144331550687130771848387666977941989898681640625;-0.1413790741896504832286751707215444184839725494384765625;0.460303224301373548055238416054635308682918548583984375]
      mask Display: e = 0.06;c1 = [120 150 230]/255;c2 = ([120 150 230]+0)/383;c3 = ([120 150 230]+128)/383;patch([0 1 1 0],[0 0 1 1],c1);patch([0 1 1 1-e 1-e 0+e],[0 0 1 1-e 0+e 0+e],c2);patch([0 0 1 1-e 0+e 0+e],[0 1 1 1-e 1-e 0+e],c3);plot([0 1 1 0 0],[0 0 1 1 0]);disp('Weights');
  "IW{1,1}(2,:)'" : Constant  Value=[-1.579381855283906954667827449156902730464935302734375;-0.33856178041791995525500169605948030948638916015625;-0.8442277384139789120354180340655148029327392578125;0.0212594351822440082167009478553154622204601764678955078125]
      mask Display: e = 0.06;c1 = [120 150 230]/255;c2 = ([120 150 230]+0)/383;c3 = ([120 150 230]+128)/383;patch([0 1 1 0],[0 0 1 1],c1);patch([0 1 1 1-e 1-e 0+e],[0 0 1 1-e 0+e 0+e],c2);patch([0 0 1 1-e 0+e 0+e],[0 1 1 1-e 1-e 0+e],c3);plot([0 1 1 0 0],[0 0 1 1 0]);disp('Weights');
  "IW{1,1}(3,:)'" : Constant  Value=[0.38376229632346581244206618066527880728244781494140625;-0.37328134764323916972017514126491732895374298095703125;0.2092431405073534589345030099138966761529445648193359375;-0.1762361278029307143366821719610015861690044403076171875]
      mask Display: e = 0.06;c1 = [120 150 230]/255;c2 = ([120 150 230]+0)/383;c3 = ([120 150 230]+128)/383;patch([0 1 1 0],[0 0 1 1],c1);patch([0 1 1 1-e 1-e 0+e],[0 0 1 1-e 0+e 0+e],c2);patch([0 0 1 1-e 0+e 0+e],[0 1 1 1-e 1-e 0+e],c3);plot([0 1 1 0 0],[0 0 1 1 0]);disp('Weights');
  "IW{1,1}(4,:)'" : Constant  Value=[-2.726931015925468049232449629926122725009918212890625;-0.61731902070469235610516989254392683506011962890625;-1.5561469263110840888231223289039917290210723876953125;0.13471390910407643470847460775985382497310638427734375]
      mask Display: e = 0.06;c1 = [120 150 230]/255;c2 = ([120 150 230]+0)/383;c3 = ([120 150 230]+128)/383;patch([0 1 1 0],[0 0 1 1],c1);patch([0 1 1 1-e 1-e 0+e],[0 0 1 1-e 0+e 0+e],c2);patch([0 0 1 1-e 0+e 0+e],[0 1 1 1-e 1-e 0+e],c3);plot([0 1 1 0 0],[0 0 1 1 0]);disp('Weights');
  "IW{1,1}(5,:)'" : Constant  Value=[-0.05662475727607456377210581877079675905406475067138671875;-1.3567365164425446710794176397030241787433624267578125;0.04612182222798731634494373565757996402680873870849609375;-0.5674886551852684757335509857512079179286956787109375]
      mask Display: e = 0.06;c1 = [120 150 230]/255;c2 = ([120 150 230]+0)/383;c3 = ([120 150 230]+128)/383;patch([0 1 1 0],[0 0 1 1],c1);patch([0 1 1 1-e 1-e 0+e],[0 0 1 1-e 0+e 0+e],c2);patch([0 0 1 1-e 0+e 0+e],[0 1 1 1-e 1-e 0+e],c3);plot([0 1 1 0 0],[0 0 1 1 0]);disp('Weights');
  Mux : Mux  Inputs=5
      mask Display: e = 0.06;c1 = [120 150 230]/255;c2 = ([120 150 230]+0)/383;c3 = ([120 150 230]+128)/383;patch([0 1 1 0],[0 0 1 1],c1);patch([0 1 1 1-e 1-e 0+e],[0 0 1 1-e 0+e 0+e],c2);patch([0 0 1 1-e 0+e 0+e],[0 1 1 1-e 1-e 0+e],c3);plot([0 1 1 0 0],[0 0 1 1 0]);disp('Mux');
  dotprod{1..5} (5 alike) : neural/Weight Functions/dotprod
  "iz{1,1}" : Outport
      mask Display: e = 0.06;c1 = [120 230 180]/255;c2 = ([120 230 180]+0)/(256+128);c3 = ([120 230 180]+128)/(256+128);patch([0 1 1 0],[0 0 1 1],c1);patch([0 1 1 1-e 1-e 0+e],[0 0 1 1-e 0+e 0+e],c2);patch([0 0 1 1-e 0+e 0+e],[0 1 1 1-e 1-e 0+e],c3);plot([0 1 1 0 0],[0 0 1 1 0]);
  wires:
  "IW{1,1}(1,:)'"/1 -> dotprod1/1
  "pd{1,1}"/1 -> dotprod1/2, dotprod2/2, dotprod3/2, dotprod4/2, dotprod5/2
  dotprod1/1 -> Mux/1
  "IW{1,1}(2,:)'"/1 -> dotprod2/1
  dotprod2/1 -> Mux/2
  "IW{1,1}(3,:)'"/1 -> dotprod3/1
  dotprod3/1 -> Mux/3
  "IW{1,1}(4,:)'"/1 -> dotprod4/1
  dotprod4/1 -> Mux/4
  "IW{1,1}(5,:)'"/1 -> dotprod5/1
  dotprod5/1 -> Mux/5
  Mux/1 -> "iz{1,1}"/1

== system XY_2mm_accelcontrol/get_plant_input/acceleration_to_I_ratio/Voltages from ML/Function Fitting Neural Network/Layer 2/Delays 1 ==
  "p{2}" : Inport  PortDimensions=5
      mask Display: e = 0.06;c1 = [120 230 180]/255;c2 = ([120 230 180]+0)/(256+128);c3 = ([120 230 180]+128)/(256+128);patch([0 1 1 0],[0 0 1 1],c1);patch([0 1 1 1-e 1-e 0+e],[0 0 1 1-e 0+e 0+e],c2);patch([0 0 1 1-e 0+e 0+e],[0 1 1 1-e 1-e 0+e],c3);plot([0 1 1 0 0],[0 0 1 1 0]);
  mux : Mux  Inputs=1
      mask Display: e = 0.06;c1 = [120 150 230]/255;c2 = ([120 150 230]+0)/383;c3 = ([120 150 230]+128)/383;patch([0 1 1 0],[0 0 1 1],c1);patch([0 1 1 1-e 1-e 0+e],[0 0 1 1-e 0+e 0+e],c2);patch([0 0 1 1-e 0+e 0+e],[0 1 1 1-e 1-e 0+e],c3);plot([0 1 1 0 0],[0 0 1 1 0]);disp('Mux')
  "pd{2,1}" : Outport
      mask Display: e = 0.06;c1 = [120 230 180]/255;c2 = ([120 230 180]+0)/(256+128);c3 = ([120 230 180]+128)/(256+128);patch([0 1 1 0],[0 0 1 1],c1);patch([0 1 1 1-e 1-e 0+e],[0 0 1 1-e 0+e 0+e],c2);patch([0 0 1 1-e 0+e 0+e],[0 1 1 1-e 1-e 0+e],c3);plot([0 1 1 0 0],[0 0 1 1 0]);
  wires:
  "p{2}"/1 -> mux/1
  mux/1 -> "pd{2,1}"/1

== system XY_2mm_accelcontrol/get_plant_input/acceleration_to_I_ratio/Voltages from ML/Function Fitting Neural Network/Layer 2/LW{2,1} ==
  "ad{2,1}" : Inport  PortDimensions=5
      mask Display: e = 0.06;c1 = [120 230 180]/255;c2 = ([120 230 180]+0)/(256+128);c3 = ([120 230 180]+128)/(256+128);patch([0 1 1 0],[0 0 1 1],c1);patch([0 1 1 1-e 1-e 0+e],[0 0 1 1-e 0+e 0+e],c2);patch([0 0 1 1-e 0+e 0+e],[0 1 1 1-e 1-e 0+e],c3);plot([0 1 1 0 0],[0 0 1 1 0]);
  "IW{2,1}(1,:)'" : Constant  Value=[-8.41948546524191243634049897082149982452392578125;-1.094337190509742985256025349372066557407379150390625;-8.8358523185672996902439990662969648838043212890625;-0.366668799998960015518179034188506193459033966064453125;-4.73035481547747860275876519153825938701629638671875]
      mask Display: e = 0.06;c1 = [120 150 230]/255;c2 = ([120 150 230]+0)/383;c3 = ([120 150 230]+128)/383;patch([0 1 1 0],[0 0 1 1],c1);patch([0 1 1 1-e 1-e 0+e],[0 0 1 1-e 0+e 0+e],c2);patch([0 0 1 1-e 0+e 0+e],[0 1 1 1-e 1-e 0+e],c3);plot([0 1 1 0 0],[0 0 1 1 0]);disp('weights');
  "IW{2,1}(2,:)'" : Constant  Value=[9.78742295100466463964039576239883899688720703125;1.273701754174963785004592864424921572208404541015625;7.9004914477829810692810497130267322063446044921875;0.57810174701958871867901734731276519596576690673828125;5.61542114311950069094336868147365748882293701171875]
      mask Display: e = 0.06;c1 = [120 150 230]/255;c2 = ([120 150 230]+0)/383;c3 = ([120 150 230]+128)/383;patch([0 1 1 0],[0 0 1 1],c1);patch([0 1 1 1-e 1-e 0+e],[0 0 1 1-e 0+e 0+e],c2);patch([0 0 1 1-e 0+e 0+e],[0 1 1 1-e 1-e 0+e],c3);plot([0 1 1 0 0],[0 0 1 1 0]);disp('weights');
  "IW{2,1}(3,:)'" : Constant  Value=[-8.7835225646644357055947693879716098308563232421875;-0.1624081142248008091666378049922059290111064910888671875;-6.07135360954028069357946151285432279109954833984375;0.019997115256658710980008919477768358774483203887939453125;-5.0263827423299378693855032906867563724517822265625]
      mask Display: e = 0.06;c1 = [120 150 230]/255;c2 = ([120 150 230]+0)/383;c3 = ([120 150 230]+128)/383;patch([0 1 1 0],[0 0 1 1],c1);patch([0 1 1 1-e 1-e 0+e],[0 0 1 1-e 0+e 0+e],c2);patch([0 0 1 1-e 0+e 0+e],[0 1 1 1-e 1-e 0+e],c3);plot([0 1 1 0 0],[0 0 1 1 0]);disp('weights');
  "IW{2,1}(4,:)'" : Constant  Value=[8.4755214194344272726766575942747294902801513671875;1.0957318445634383063946870606741867959499359130859375;8.86393875358810845455082016997039318084716796875;0.363765057531977131777267686629784293472766876220703125;4.7702460563195785425705253146588802337646484375]
      mask Display: e = 0.06;c1 = [120 150 230]/255;c2 = ([120 150 230]+0)/383;c3 = ([120 150 230]+128)/383;patch([0 1 1 0],[0 0 1 1],c1);patch([0 1 1 1-e 1-e 0+e],[0 0 1 1-e 0+e 0+e],c2);patch([0 0 1 1-e 0+e 0+e],[0 1 1 1-e 1-e 0+e],c3);plot([0 1 1 0 0],[0 0 1 1 0]);disp('weights');
  "IW{2,1}(5,:)'" : Constant  Value=[-9.7245431489428231230931487516500055789947509765625;-1.2706136829687666445209970333962701261043548583984375;-7.8414256254865222217631526291370391845703125;-0.5663485516887032389377054641954600811004638671875;-5.58997080669033419297875298070721328258514404296875]
      mask Display: e = 0.06;c1 = [120 150 230]/255;c2 = ([120 150 230]+0)/383;c3 = ([120 150 230]+128)/383;patch([0 1 1 0],[0 0 1 1],c1);patch([0 1 1 1-e 1-e 0+e],[0 0 1 1-e 0+e 0+e],c2);patch([0 0 1 1-e 0+e 0+e],[0 1 1 1-e 1-e 0+e],c3);plot([0 1 1 0 0],[0 0 1 1 0]);disp('weights');
  "IW{2,1}(6,:)'" : Constant  Value=[8.853411540722515127299629966728389263153076171875;0.1702991597133139134445656281968695111572742462158203125;6.1297048497102988307005944079719483852386474609375;-0.02119364708076641734546541329109459184110164642333984375;5.0636234193474312093030675896443426609039306640625]
      mask Display: e = 0.06;c1 = [120 150 230]/255;c2 = ([120 150 230]+0)/383;c3 = ([120 150 230]+128)/383;patch([0 1 1 0],[0 0 1 1],c1);patch([0 1 1 1-e 1-e 0+e],[0 0 1 1-e 0+e 0+e],c2);patch([0 0 1 1-e 0+e 0+e],[0 1 1 1-e 1-e 0+e],c3);plot([0 1 1 0 0],[0 0 1 1 0]);disp('weights');
  Mux : Mux  Inputs=6
      mask Display: e = 0.06;c1 = [120 150 230]/255;c2 = ([120 150 230]+0)/383;c3 = ([120 150 230]+128)/383;patch([0 1 1 0],[0 0 1 1],c1);patch([0 1 1 1-e 1-e 0+e],[0 0 1 1-e 0+e 0+e],c2);patch([0 0 1 1-e 0+e 0+e],[0 1 1 1-e 1-e 0+e],c3);plot([0 1 1 0 0],[0 0 1 1 0]);disp('Mux');
  dotprod{1..6} (6 alike) : neural/Weight Functions/dotprod
  "lz{2,1}" : Outport
      mask Display: e = 0.06;c1 = [120 230 180]/255;c2 = ([120 230 180]+0)/(256+128);c3 = ([120 230 180]+128)/(256+128);patch([0 1 1 0],[0 0 1 1],c1);patch([0 1 1 1-e 1-e 0+e],[0 0 1 1-e 0+e 0+e],c2);patch([0 0 1 1-e 0+e 0+e],[0 1 1 1-e 1-e 0+e],c3);plot([0 1 1 0 0],[0 0 1 1 0]);
  wires:
  "IW{2,1}(1,:)'"/1 -> dotprod1/1
  "ad{2,1}"/1 -> dotprod1/2, dotprod2/2, dotprod3/2, dotprod4/2, dotprod5/2, dotprod6/2
  dotprod1/1 -> Mux/1
  "IW{2,1}(2,:)'"/1 -> dotprod2/1
  dotprod2/1 -> Mux/2
  "IW{2,1}(3,:)'"/1 -> dotprod3/1
  dotprod3/1 -> Mux/3
  "IW{2,1}(4,:)'"/1 -> dotprod4/1
  dotprod4/1 -> Mux/4
  "IW{2,1}(5,:)'"/1 -> dotprod5/1
  dotprod5/1 -> Mux/5
  "IW{2,1}(6,:)'"/1 -> dotprod6/1
  dotprod6/1 -> Mux/6
  Mux/1 -> "lz{2,1}"/1

== matlab function XY_2mm_accelcontrol/get_plant_input/Z_1dctrl/PID-Vertical/max(0,|u|-1mm) ==
  data: u input; y output
function y = max_0_abs_u_minus_1mm(u)

y = max(0,abs(u)-0.0001);

== matlab function XY_2mm_accelcontrol/Input parameters/Acceleration input/MATLAB Function ==
  data: unit_mode input; x_acc_mmss output; x_acc input; y_acc input; y_acc_mmss output; errorflag output
function [x_acc_mmss,y_acc_mmss,errorflag]= acc_unit_converter(unit_mode,x_acc,y_acc)
% User can specify desired acceleration for magnet
% (units: "mm/s/s" or "micrometre/s/s")

errorflag = 0;

% NOTE: Unit modes are:
% 1 - mm/s/s
% 2 - micrometre/s/s
if unit_mode==1
    units_to_mmss = 1;
elseif unit_mode==2
    units_to_mmss = 1/1000;
else
    % (TEMP?) Assume that the user wants mm/s/s
    units_to_mmss = 1;
end

% Apply new units
x_acc_mmss = x_acc * units_to_mmss;
y_acc_mmss = y_acc * units_to_mmss;

== matlab function XY_2mm_accelcontrol/Input parameters/Magnet Specs/Magnet Physical Specs ==
  data: unit_mode input; diameter input; height input; diameter_m output; height_m output; mass_g output; B_r output; mass input; magnet_remanence_t input; errorflag output
function [diameter_m,height_m,mass_g,B_r,errorflag]= mag_specs(unit_mode,diameter,height,mass,magnet_remanence_t)
% User can specify parameters for cylindrical magnets: diameter, height 
% (units: "in" or "cm" or "mm" or "m"), mass, and either remanent B-field
% (in T or G) or magnetic dipole moment (in N*m/T, aka A*m^2).
% TO IMPLEMENT: Ring magnets!

errorflag = 0;

%%% DIMENSIONS %%%
% Dimensions, in m
% NOTE: Unit modes are:
% 1 - m
% 2 - cm
% 3 - mm
% 4 - in
if unit_mode==1
    units_to_m = 1;
elseif unit_mode==2
    units_to_m = 0.01;
elseif unit_mode==3
    units_to_m = 0.001;
elseif unit_mode==4
    units_to_m = 0.0254;
else
    % (TEMP?) Assume that the user wants metres
    units_to_m = 1;
end

% Dimensions
% if isnan(diameter)
%     diameter = diameter_detect;
% end
% if isnan(diameter_detect)
%     diameter_detect = diameter;
% end
% if isnan(height)
%     height = height_detect;
% end
% if isnan(height_detect)
%     height_detect = height;
% end
diameter_m = diameter * units_to_m;
height_m = height * units_to_m;
mass_g = mass;

%%% MAG FIELD STUFF %%%
% Mag field info (Br in Gauss or T)
if magnet_remanence_t > 1000
    % Assumes a remanence field value based on the material, in Gauss.
    % For example, an N52 magnet has 14800G, and Xiaodong's now-battered
    % magnet has 12900G.
    B_r = magnet_remanence_t / 10000;
else
    % Assumes a remanence field value based on the material, in T.
    % For example, an N52 magnet has 1.48T, and Xiaodong's now-battered
    % magnet has 1.29T.
    B_r = magnet_remanence_t / 1;
end

% (!!!!) CREATE CHART FOR CONVERSION FROM Nxx FORMAT TO REMANENCE IN T

% K&J SPECS:
%     % Assumes a grade was inputted as a string-- N52, N42, etc!
%     if lower(magfield_grade_t)=="n52"
%         B_r = 1.48;
%     elseif lower(magfield_grade_t)=="n50"
%         B_r = 1.45;
%     elseif lower(magfield_grade_t)=="n48"
%         B_r = 1.42;
%     elseif lower(magfield_grade_t)=="n45"
%         B_r = 1.35;
%     elseif lower(magfield_grade_t)=="n42"
%         B_r = 1.32;
%     elseif lower(magfield_grade_t)=="n40"
%         B_r = 1.29;
%     elseif lower(magfield_grade_t)=="n35"
%         B_r = 1.21;
%     else
%         % SHOULD NEVER HAPPEN
%         B_r = 1.48;
%         errorflag = 1;
%     end
% APPLIEDMAGNETS SPECS:
%     % Assumes a grade was inputted as a string-- N52, N42, etc!
%     if lower(magfield_grade_t)=="n52"
%         B_r = 1.48;
%     elseif lower(magfield_grade_t)=="n50"
%         B_r = 1.45;
%     elseif lower(magfield_grade_t)=="n48"
%         B_r = 1.42;
%     elseif lower(magfield_grade_t)=="n45"
%         B_r = 1.38 (rarely 1.35);
%     elseif lower(magfield_grade_t)=="n42"
%         B_r = 1.32;
%     elseif lower(magfield_grade_t)=="n40"
%         B_r = 1.29;
%     else
%         % SHOULD NEVER HAPPEN
%         B_r = 1.48;
%         errorflag = 1;
%     end
% 
% 
%

== matlab function XY_2mm_accelcontrol/get_plant_input/choose_Z_d_temp/recovery_mode_toggle ==
  data: isstable input; recovery_mode output; isconverged input; recovery_mode input
function recovery_mode = recovery_mode_toggle(isstable,isconverged, recovery_mode)
% "recovery_mode" takes the value of one of the following:
%       0: 'safe' (default) : Default behaviour; dz_max is set to its max.
%       1: 'panic' : Magnet has left the workspace entirely.
%       2: 'recovery' : Instability detected. 

%     % Choose recovery mode
    if ~isstable
        % If unstable, then enable 'recovery' mode.
        recovery_mode = 2;
    else
        if recovery_mode==0
            % Do nothing.
%         elseif recovery_mode==2 && isconverged_Zdtemp_heldforXtime
%             % If it converges during 'panic' mode, then 'recovery' mode can
%             % safely be enabled.
%             if isconverged_Zdtemp
%                 recovery_mode = 2;
%             end
        elseif recovery_mode==2
            % If it converges onto z_d_true during 'recovery' mode, then
            % it's safe to go back to 'safe' mode.
            if isconverged
                recovery_mode = 0;
            end
        end
    end


end
